simulink model "Symmetry_Inverter_imagined"  (Simulink 8.1)
settings: Solver=ode23t  StartTime=0.0  StopTime=tfin  RelTol=1e-4
values from neighbouring files (symbols this model uses):
  amp_feedback_saturation = 400    [Symmetry_ini_COPY.m]
  Butterworth_filter_order = 8    [Symmetry_ini_COPY.m]
  initial_value = [0.00,0.00,0.00,                  0,0,0]    [Symmetry_ini_COPY.m]
  k_symmetrcal_gain = 1e1    (= 10)    [Symmetry_ini_COPY.m]
  L_Network = [3.185e-3, 3.185e-3, 3.185e-3, 3.185e-3]    [Symmetry_ini_COPY.m]
  L_Source = [3.185e-3, 3.185e-3, 3.185e-3]    [Symmetry_ini_COPY.m]
  Load_R = [50,50,50]    [Symmetry_ini_COPY.m]
  Load_RL = [35.35,   35.35,   35.35;                   0.1125,  0.1125,  0.1125]    [Symmetry_ini_COPY.m]
  NetworkBreaker = [1e5,1e5,1e5,1e5]    [Symmetry_ini_COPY.m]
  P_gain = 5e-5    (= 5e-05)    [Symmetry_ini_COPY.m]
  phase_feedback_saturation = pi    (= 3.14159265359)    [Symmetry_ini_COPY.m]
  Phase_Source = [0,-2/3*pi,-4/3*pi]    [Symmetry_ini_COPY.m]
  PowerGain = [1e-5,1e-5,0]    [Symmetry_ini_COPY.m]
  PV_Power_Capacity = 5e3    (= 5000)    [Symmetry_ini_COPY.m]
  R_Source = [0.4, 0.4, 0.4]    [Symmetry_ini_COPY.m]
  sample = 10e-5    (= 0.0001)    [Symmetry_ini_COPY.m]    (also in animated_norms.m)
  Source_Frequency = [50,50,50]    [Symmetry_ini_COPY.m]
  Start_Control = 0.5    [Symmetry_ini_COPY.m]
  step_size = [1,1,1,                  0.08,0.08,0.08]    [Symmetry_ini_COPY.m]
  test_step = [0.5,0.5,0.5,                  0.02,0.02,0.02]    [Symmetry_ini_COPY.m]
  TransformerBreaker = [1e5,1e5,1e5;                     1e5,1e5,1e5]    [Symmetry_ini_COPY.m]
  Urms_Source = [230,230,230]    [Symmetry_ini_COPY.m]
undefined symbols (not defined in the file or in its folder): Capacitive_Load_RC, START_Load, Wire_resistence
libraries: powerlib x55, simulink x18, dspsigops x10, commsequence2 x6, powerlib_extras x6, dspxfrm3 x3, dsparch4 x3
(part 1 of 2)
settings Model: Creator=gorbep  LastModifiedBy=Neukirchner László
settings SolverCC: ZeroCrossAlgorithm=Adaptive  AlgebraicLoopSolver=LineSearch  SolverResetMethod=Robust
settings DataIOCC: SignalLoggingSaveFormat=Dataset
settings OptimizationCC: ExpressionDepthLimit=128  SimCompilerOptimization=On
settings DebuggingCC: UnderspecifiedInitializationDetection=Simplified  IgnoredZcDiagnostic=none  FcnCallInpInsideContextMsg=EnableAllAsError  StateNameClashWarn=none
settings GRTTargetCC: CodeReplacementLibrary=None  CombineOutputUpdateFcns=on  CPPClassGenCompliant=on  GRTInterface=off

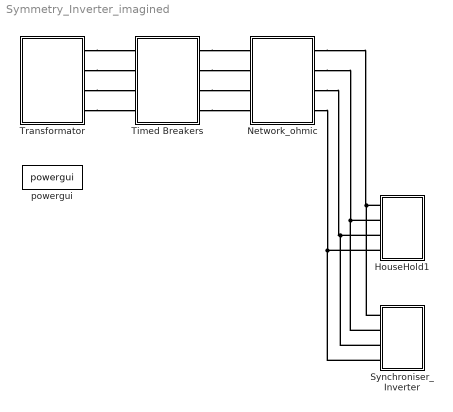
== system Symmetry_Inverter_imagined ==
  "HouseHold1 " : Subsystem
  Network_ohmic : Subsystem
  Synchroniser_Inverter : Subsystem
  Timed Breakers : Subsystem
  Transformator : Subsystem
  powergui : powerlib/powergui  SimulationMode=Continuous  SolverType=Tustin  SampleTime=50e-6  frequency=60  SPID=off  DisableSnubberDevices=off  DisableRonSwitches=off  DisableVfSwitches=off  SwTol=0  Interpol=off  DisplayEquations=off  frequencyindice=0  Pbase=100e6  ErrMax=1e-4  Iterations=50  UnitsV=kV  UnitsW=MW  FunctionMessages=off  echomessages=off  HookPort=off  EnableUseOfTLC=off  x0status=blocks  RestoreLinks=warning  ResistiveCurrentMeasurement=off  Frange=[0:2:500]  Ylog=off  Xlog=on  ShowGrid=off  save=off  variable=ZData  structure=0  ZoomFFT=on  StartTime=0.0  cycles=1  DisplayStyle=1  fundamental=60  FreqAxis=off  MaxFrequency=1000  frequencyindicesteady=1  RmsSteady=1  display=off  Ts=0  methode=off
  connections:
  Transformator/RConn1 -- Timed Breakers/LConn1
  Transformator/RConn2 -- Timed Breakers/LConn2
  Transformator/RConn3 -- Timed Breakers/LConn3
  Transformator/RConn4 -- Timed Breakers/LConn4
  Timed Breakers/RConn1 -- Network_ohmic/LConn1
  Timed Breakers/RConn3 -- Network_ohmic/LConn3
  Timed Breakers/RConn4 -- Network_ohmic/LConn4
  Timed Breakers/RConn2 -- Network_ohmic/LConn2
  Network_ohmic/RConn1 -- Synchroniser_Inverter/LConn1 -- "HouseHold1 "/LConn1
  Network_ohmic/RConn2 -- Synchroniser_Inverter/LConn2 -- "HouseHold1 "/LConn2
  Network_ohmic/RConn3 -- Synchroniser_Inverter/LConn3 -- "HouseHold1 "/LConn3
  Network_ohmic/RConn4 -- Synchroniser_Inverter/LConn4 -- "HouseHold1 "/LConn4

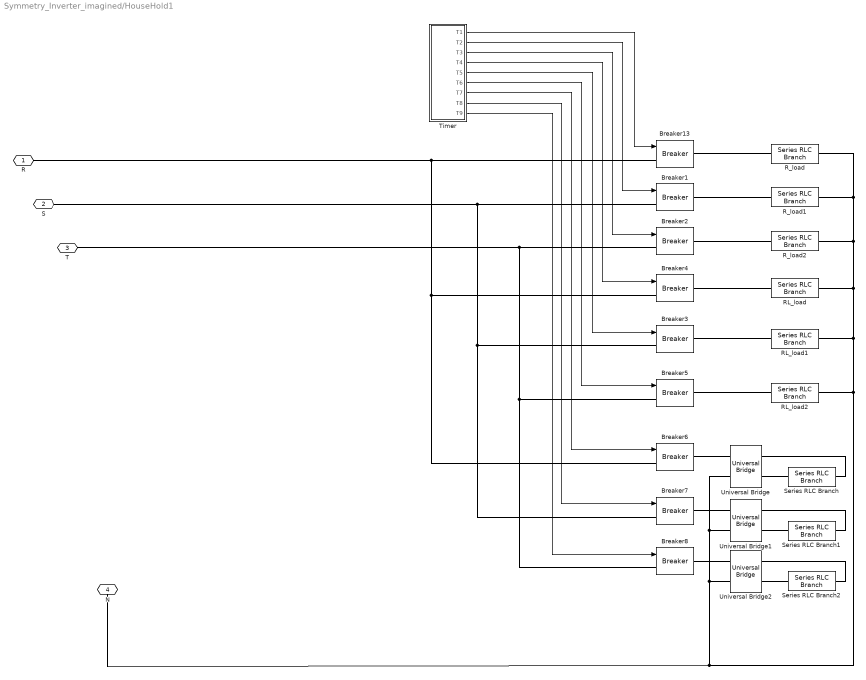
== system Symmetry_Inverter_imagined/HouseHold1  ==
  Breaker{1..8,13} (9 alike) : powerlib/Elements/Breaker  BreakerResistance=0.01  InitialState=0  SnubberResistance=1e7  SnubberCapacitance=inf  SwitchingTimes="[ 1/60  5/60 ]"  External=on  Measurements=None  MoreParameters=off  NoBreakLoop=off
  RL_load : powerlib/Elements/Series RLC Branch  LConnTagsString=__new0  RConnTagsString=__new0  BranchType=RL  Resistance=Load_RL(1,1)  Inductance=Load_RL(2,1)  SetiL0=off  InitialCurrent=0  Capacitance=1.0  Setx0=off  InitialVoltage=0  Measurements=None
  RL_load1 : powerlib/Elements/Series RLC Branch  LConnTagsString=__new0  RConnTagsString=__new0  BranchType=RL  Resistance=Load_RL(1,2)  Inductance=Load_RL(2,2)  SetiL0=off  InitialCurrent=0  Capacitance=1.0  Setx0=off  InitialVoltage=0  Measurements=None
  RL_load2 : powerlib/Elements/Series RLC Branch  LConnTagsString=__new0  RConnTagsString=__new0  BranchType=RL  Resistance=Load_RL(1,3)  Inductance=Load_RL(2,3)  SetiL0=off  InitialCurrent=0  Capacitance=1.0  Setx0=off  InitialVoltage=0  Measurements=None
  R_load : powerlib/Elements/Series RLC Branch  LConnTagsString=__new0  RConnTagsString=__new0  BranchType=R  Resistance=Load_R(1)  Inductance=0.003185  SetiL0=off  InitialCurrent=0  Capacitance=1.0  Setx0=off  InitialVoltage=0  Measurements=None
  R_load1 : powerlib/Elements/Series RLC Branch  LConnTagsString=__new0  RConnTagsString=__new0  BranchType=R  Resistance=Load_R(2)  Inductance=0.003185  SetiL0=off  InitialCurrent=0  Capacitance=1.0  Setx0=off  InitialVoltage=0  Measurements=None
  R_load2 : powerlib/Elements/Series RLC Branch  LConnTagsString=__new0  RConnTagsString=__new0  BranchType=R  Resistance=Load_R(3)  Inductance=0.003185  SetiL0=off  InitialCurrent=0  Capacitance=1.0  Setx0=off  InitialVoltage=0  Measurements=None
  Series RLC Branch : powerlib/Elements/Series RLC Branch  LConnTagsString=__new0  RConnTagsString=__new0  BranchType=RC  Resistance=Capacitive_Load_RC(1,1)  Inductance=1e-3  SetiL0=off  InitialCurrent=0  Capacitance=Capacitive_Load_RC(2,1)  Setx0=off  InitialVoltage=0  Measurements=None
  Series RLC Branch1 : powerlib/Elements/Series RLC Branch  LConnTagsString=__new0  RConnTagsString=__new0  BranchType=RC  Resistance=Capacitive_Load_RC(1,2)  Inductance=1e-3  SetiL0=off  InitialCurrent=0  Capacitance=Capacitive_Load_RC(2,2)  Setx0=off  InitialVoltage=0  Measurements=None
  Series RLC Branch2 : powerlib/Elements/Series RLC Branch  LConnTagsString=__new0  RConnTagsString=__new0  BranchType=RC  Resistance=Capacitive_Load_RC(1,3)  Inductance=1e-3  SetiL0=off  InitialCurrent=0  Capacitance=Capacitive_Load_RC(2,3)  Setx0=off  InitialVoltage=0  Measurements=None
  Timer : Subsystem
  Universal Bridge : powerlib/Power Electronics/Universal Bridge  Arms=2  SnubberResistance=1e5  SnubberCapacitance=inf  Device=Diodes  Ron=1e-3  Lon=0  ForwardVoltages="[  0  0  ]"  ForwardVoltage=0.8  GTOparameters=[ 10e-6 , 20e-6 ]  IGBTparameters=[ 1e-6 , 2e-6 ]  Measurements=None  Measurements_2=None  converterType=Rectifier
  Universal Bridge1 : powerlib/Power Electronics/Universal Bridge  Arms=2  SnubberResistance=1e5  SnubberCapacitance=inf  Device=Diodes  Ron=1e-3  Lon=0  ForwardVoltages="[  0  0  ]"  ForwardVoltage=0.8  GTOparameters=[ 10e-6 , 20e-6 ]  IGBTparameters=[ 1e-6 , 2e-6 ]  Measurements=None  Measurements_2=None  converterType=Rectifier
  Universal Bridge2 : powerlib/Power Electronics/Universal Bridge  Arms=2  SnubberResistance=1e5  SnubberCapacitance=inf  Device=Diodes  Ron=1e-3  Lon=0  ForwardVoltages="[  0  0  ]"  ForwardVoltage=0.8  GTOparameters=[ 10e-6 , 20e-6 ]  IGBTparameters=[ 1e-6 , 2e-6 ]  Measurements=None  Measurements_2=None  converterType=Rectifier
  R : PMIOPort  Port=1  Side=Left
  S : PMIOPort  Port=2  Side=Left
  T : PMIOPort  Port=3  Side=Left
  N : PMIOPort  Port=4  Side=Left
  wires:
  Timer/1(T1) -> Breaker13/1
  Timer/2(T2) -> Breaker1/1
  Timer/3(T3) -> Breaker2/1
  Timer/4(T4) -> Breaker4/1
  Timer/5(T5) -> Breaker3/1
  Timer/6(T6) -> Breaker5/1
  Timer/7(T7) -> Breaker6/1
  Timer/8(T8) -> Breaker7/1
  Timer/9(T9) -> Breaker8/1
  connections:
  R_load2/LConn1 -- Breaker2/RConn1
  R_load1/LConn1 -- Breaker1/RConn1
  Breaker13/RConn1 -- R_load/LConn1
  RL_load1/RConn1 -- RL_load/RConn1 -- R_load/RConn1 -- R_load1/RConn1 -- R_load2/RConn1 -- N/RConn1 -- Universal Bridge2/LConn2 -- Universal Bridge1/LConn2 -- Universal Bridge/LConn2 -- RL_load2/RConn1
  Breaker4/RConn1 -- RL_load/LConn1
  RL_load2/LConn1 -- Breaker5/RConn1
  RL_load1/LConn1 -- Breaker3/RConn1
  Breaker6/RConn1 -- Universal Bridge/LConn1
  Universal Bridge/RConn1 -- Series RLC Branch/LConn1
  Universal Bridge/RConn2 -- Series RLC Branch/RConn1
  Breaker7/RConn1 -- Universal Bridge1/LConn1
  Universal Bridge1/RConn2 -- Series RLC Branch1/RConn1
  Universal Bridge1/RConn1 -- Series RLC Branch1/LConn1
  Universal Bridge2/RConn2 -- Series RLC Branch2/RConn1
  Breaker8/RConn1 -- Universal Bridge2/LConn1
  Universal Bridge2/RConn1 -- Series RLC Branch2/LConn1
  Breaker6/LConn1 -- Breaker4/LConn1 -- R/RConn1 -- Breaker13/LConn1
  Breaker7/LConn1 -- Breaker3/LConn1 -- S/RConn1 -- Breaker1/LConn1
  Breaker8/LConn1 -- Breaker5/LConn1 -- T/RConn1 -- Breaker2/LConn1

== system Symmetry_Inverter_imagined/Network_ohmic ==
  Transf-L  Line -R1 : powerlib/Elements/Series RLC Branch  LConnTagsString=__new0  RConnTagsString=__new0  BranchType=R  Resistance=Wire_resistence  Inductance=L_Network(1)  SetiL0=off  InitialCurrent=0  Capacitance=1.0  Setx0=off  InitialVoltage=0  Measurements=None
  Transf-L  Line -R2 : powerlib/Elements/Series RLC Branch  LConnTagsString=__new0  RConnTagsString=__new0  BranchType=R  Resistance=Wire_resistence  Inductance=L_Network(2)  SetiL0=off  InitialCurrent=0  Capacitance=1.0  Setx0=off  InitialVoltage=0  Measurements=None
  Transf-L  Line -R3 : powerlib/Elements/Series RLC Branch  LConnTagsString=__new0  RConnTagsString=__new0  BranchType=R  Resistance=Wire_resistence  Inductance=L_Network(3)  SetiL0=off  InitialCurrent=0  Capacitance=1.0  Setx0=off  InitialVoltage=0  Measurements=None
  Transf-L  Line -R9 : powerlib/Elements/Series RLC Branch  LConnTagsString=__new0  RConnTagsString=__new0  BranchType=R  Resistance=Wire_resistence  Inductance=L_Network(4)  SetiL0=off  InitialCurrent=0  Capacitance=1.0  Setx0=off  InitialVoltage=0  Measurements=None
  R : PMIOPort  Port=1  Side=Left
  U : PMIOPort  Port=2  Side=Right
  S : PMIOPort  Port=3  Side=Left
  V : PMIOPort  Port=4  Side=Right
  T : PMIOPort  Port=5  Side=Left
  W : PMIOPort  Port=6  Side=Right
  N : PMIOPort  Port=7  Side=Left
  n : PMIOPort  Port=8  Side=Right
  connections:
  U/RConn1 -- Transf-L  Line -R1/RConn1
  V/RConn1 -- Transf-L  Line -R2/RConn1
  W/RConn1 -- Transf-L  Line -R3/RConn1
  Transf-L  Line -R3/LConn1 -- T/RConn1
  Transf-L  Line -R2/LConn1 -- S/RConn1
  R/RConn1 -- Transf-L  Line -R1/LConn1
  Transf-L  Line -R9/LConn1 -- N/RConn1
  n/RConn1 -- Transf-L  Line -R9/RConn1

== system Symmetry_Inverter_imagined/Synchroniser_Inverter ==
  Calculate_Norms : Subsystem
  Current Control : Subsystem
  NORM : Scope
      settings: ShowLegends=on  YMin=137464  YMax=137464  SaveName=ScopeData2
  Terminator{,1..5} (6 alike) : Terminator
  R : PMIOPort  Port=1  Side=Left
  S : PMIOPort  Port=2  Side=Left
  T : PMIOPort  Port=3  Side=Left
  N : PMIOPort  Port=4  Side=Left
  wires:
  Calculate_Norms/1(REG) -> Terminator/1
  Calculate_Norms/6(GEO) -> NORM/1, Current Control/1(NORM)
  Calculate_Norms/8(ANG) -> Current Control/2(ANG)
  Calculate_Norms/2(VEC_OLD) -> Terminator1/1
  Calculate_Norms/4(VEC_OLD_MEAN) -> Terminator3/1
  Calculate_Norms/7(GEO_MEAN) -> Terminator5/1
  Calculate_Norms/5(VEC_NEW_MEAN) -> Terminator4/1
  Calculate_Norms/3(VEC_NEW) -> Terminator2/1
  connections:
  R/RConn1 -- Current Control/RConn1 -- Calculate_Norms/LConn1
  S/RConn1 -- Current Control/RConn2 -- Calculate_Norms/LConn2
  T/RConn1 -- Current Control/RConn3 -- Calculate_Norms/LConn3
  N/RConn1 -- Current Control/RConn4 -- Calculate_Norms/LConn4

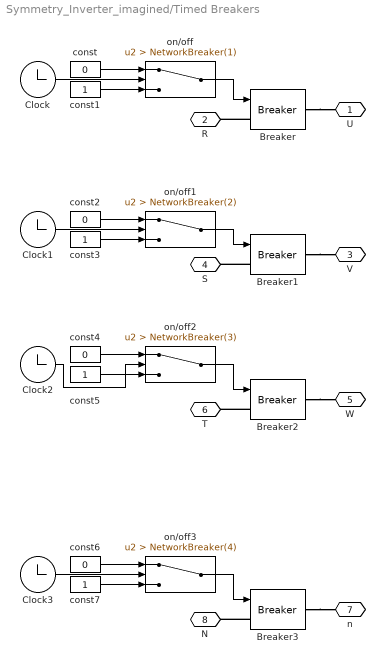
== system Symmetry_Inverter_imagined/Timed Breakers ==
  Breaker{,1..3} (4 alike) : powerlib/Elements/Breaker  BreakerResistance=0.01  InitialState=0  SnubberResistance=1e6  SnubberCapacitance=inf  SwitchingTimes="[1/60  5/60]"  External=on  Measurements=None  MoreParameters=on  NoBreakLoop=off
  Clock{,1..3} (4 alike) : Clock
      settings: Decimation=CLK
  const{,2,4,6} (4 alike) : Constant  Value=0
  const{1,3,5,7} (4 alike) : Constant
  on/off : Switch  Criteria=u2 > Threshold  Threshold=NetworkBreaker(1)
  on/off1 : Switch  Criteria=u2 > Threshold  Threshold=NetworkBreaker(2)
  on/off2 : Switch  Criteria=u2 > Threshold  Threshold=NetworkBreaker(3)
  on/off3 : Switch  Criteria=u2 > Threshold  Threshold=NetworkBreaker(4)
  U : PMIOPort  Port=1  Side=Right
  R : PMIOPort  Port=2  Side=Left
  V : PMIOPort  Port=3  Side=Right
  S : PMIOPort  Port=4  Side=Left
  W : PMIOPort  Port=5  Side=Right
  T : PMIOPort  Port=6  Side=Left
  n : PMIOPort  Port=7  Side=Right
  N : PMIOPort  Port=8  Side=Left
  wires:
  const/1 -> on/off/1
  const1/1 -> on/off/3
  Clock/1 -> on/off/2
  on/off/1 -> Breaker/1
  const2/1 -> on/off1/1
  const3/1 -> on/off1/3
  Clock1/1 -> on/off1/2
  const4/1 -> on/off2/1
  const5/1 -> on/off2/3
  Clock2/1 -> on/off2/2
  const6/1 -> on/off3/1
  const7/1 -> on/off3/3
  Clock3/1 -> on/off3/2
  on/off1/1 -> Breaker1/1
  on/off2/1 -> Breaker2/1
  on/off3/1 -> Breaker3/1
  connections:
  Breaker/RConn1 -- U/RConn1
  Breaker/LConn1 -- R/RConn1
  Breaker1/RConn1 -- V/RConn1
  Breaker1/LConn1 -- S/RConn1
  Breaker3/RConn1 -- n/RConn1
  Breaker3/LConn1 -- N/RConn1
  Breaker2/RConn1 -- W/RConn1
  Breaker2/LConn1 -- T/RConn1

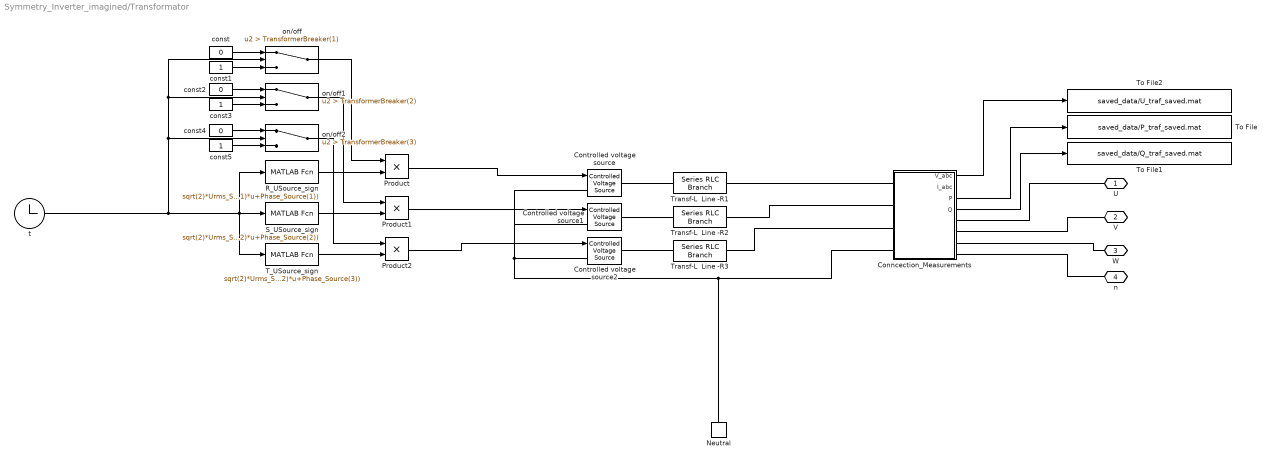
== system Symmetry_Inverter_imagined/Transformator ==
  " R_USource_sign" : MATLABFcn  MATLABFcn=sqrt(2)*Urms_Source(1)*sin(2*pi*Source_Frequency(1)*u+Phase_Source(1))  SampleTime=sample
  " S_USource_sign" : MATLABFcn  MATLABFcn=sqrt(2)*Urms_Source(2)*sin(2*pi*Source_Frequency(2)*u+Phase_Source(2))  SampleTime=sample
  " T_USource_sign" : MATLABFcn  MATLABFcn=sqrt(2)*Urms_Source(3)*sin(2*pi*Source_Frequency(2)*u+Phase_Source(3))  SampleTime=sample
  Conncection_Measurements : Subsystem
  Controlled voltage source : powerlib/Electrical Sources/Controlled Voltage Source  Initialize=off  Source_Type=AC  Amplitude=0  Phase=0  Frequency=0  Measurements=None
  Controlled voltage source1 : powerlib/Electrical Sources/Controlled Voltage Source  Initialize=off  Source_Type=AC  Amplitude=0  Phase=0  Frequency=0  Measurements=None
  Controlled voltage source2 : powerlib/Electrical Sources/Controlled Voltage Source  Initialize=off  Source_Type=AC  Amplitude=0  Phase=0  Frequency=0  Measurements=None
  Neutral : powerlib/Elements/Neutral  LConnTagsString=a  NodeNumber=10
  Product : Product
  Product1 : Product
  Product2 : Product
  To File : ToFile  Filename=saved_data/P_traf_saved.mat  MatrixName=P_traf_saved  SaveFormat=Timeseries  SampleTime=sample
  To File1 : ToFile  Filename=saved_data/Q_traf_saved.mat  MatrixName=Q_traf_saved  SaveFormat=Timeseries  SampleTime=sample
  To File2 : ToFile  Filename=saved_data/U_traf_saved.mat  MatrixName=U_traf_saved  SaveFormat=Timeseries  SampleTime=sample
  Transf-L  Line -R1 : powerlib/Elements/Series RLC Branch  LConnTagsString=__new0  RConnTagsString=__new0  BranchType=RL  Resistance=R_Source(1)  Inductance=L_Source(1)  SetiL0=off  InitialCurrent=0  Capacitance=1.0  Setx0=off  InitialVoltage=0  Measurements=None
  Transf-L  Line -R2 : powerlib/Elements/Series RLC Branch  LConnTagsString=__new0  RConnTagsString=__new0  BranchType=RL  Resistance=R_Source(2)  Inductance=L_Source(2)  SetiL0=off  InitialCurrent=0  Capacitance=1.0  Setx0=off  InitialVoltage=0  Measurements=None
  Transf-L  Line -R3 : powerlib/Elements/Series RLC Branch  LConnTagsString=__new0  RConnTagsString=__new0  BranchType=RL  Resistance=R_Source(3)  Inductance=L_Source(3)  SetiL0=off  InitialCurrent=0  Capacitance=1.0  Setx0=off  InitialVoltage=0  Measurements=None
  const : Constant  Value=0
  const1 : Constant
  const2 : Constant  Value=0
  const3 : Constant
  const4 : Constant  Value=0
  const5 : Constant
  on/off : Switch  Criteria=u2 > Threshold  Threshold=TransformerBreaker(1)
  on/off1 : Switch  Criteria=u2 > Threshold  Threshold=TransformerBreaker(2)
  on/off2 : Switch  Criteria=u2 > Threshold  Threshold=TransformerBreaker(3)
  t : Clock
      settings: Decimation=CLK
  U : PMIOPort  Port=1  Side=Right
  V : PMIOPort  Port=2  Side=Right
  W : PMIOPort  Port=3  Side=Right
  n : PMIOPort  Port=4  Side=Right
  wires:
  Conncection_Measurements/3(P) -> To File/1
  Conncection_Measurements/4(Q) -> To File1/1
  Conncection_Measurements/1(V_abc) -> To File2/1
  const/1 -> on/off/1
  const1/1 -> on/off/3
  t/1 -> " R_USource_sign"/1, " T_USource_sign"/1, " S_USource_sign"/1, on/off1/2, on/off/2, on/off2/2
  const2/1 -> on/off1/1
  const3/1 -> on/off1/3
  const4/1 -> on/off2/1
  const5/1 -> on/off2/3
  " T_USource_sign"/1 -> Product2/2
  " S_USource_sign"/1 -> Product1/2
  " R_USource_sign"/1 -> Product/2
  on/off/1 -> Product/1
  on/off1/1 -> Product1/1
  on/off2/1 -> Product2/1
  Product/1 -> Controlled voltage source/1
  Product1/1 -> Controlled voltage source1/1
  Product2/1 -> Controlled voltage source2/1
  connections:
  Neutral/LConn1 -- Conncection_Measurements/LConn4 -- Controlled voltage source/LConn1 -- Controlled voltage source1/LConn1 -- Controlled voltage source2/LConn1
  Transf-L  Line -R2/LConn1 -- Controlled voltage source1/RConn1
  Transf-L  Line -R3/LConn1 -- Controlled voltage source2/RConn1
  Transf-L  Line -R1/LConn1 -- Controlled voltage source/RConn1
  Conncection_Measurements/LConn1 -- Transf-L  Line -R1/RConn1
  Conncection_Measurements/LConn2 -- Transf-L  Line -R2/RConn1
  Conncection_Measurements/LConn3 -- Transf-L  Line -R3/RConn1
  U/RConn1 -- Conncection_Measurements/RConn1
  V/RConn1 -- Conncection_Measurements/RConn2
  W/RConn1 -- Conncection_Measurements/RConn3
  n/RConn1 -- Conncection_Measurements/RConn4

== system Symmetry_Inverter_imagined/HouseHold1 /Timer ==
  Clock : Clock
      settings: Decimation=CLK
  const : Constant
  const1 : Constant  Value=0
  on/off : Switch  Criteria=u2 > Threshold  Threshold=START_Load(1,1)
  on/off1 : Switch  Criteria=u2 > Threshold  Threshold=START_Load(1,2)
  on/off2 : Switch  Criteria=u2 > Threshold  Threshold=START_Load(1,3)
  on/off3 : Switch  Criteria=u2 > Threshold  Threshold=START_Load(2,1)
  on/off4 : Switch  Criteria=u2 > Threshold  Threshold=START_Load(2,2)
  on/off5 : Switch  Criteria=u2 > Threshold  Threshold=START_Load(2,3)
  on/off6 : Switch  Criteria=u2 > Threshold  Threshold=START_Load(3,1)
  on/off7 : Switch  Criteria=u2 > Threshold  Threshold=START_Load(3,2)
  on/off8 : Switch  Criteria=u2 > Threshold  Threshold=START_Load(3,3)
  T1 : Outport
  T2 : Outport  Port=2
  T3 : Outport  Port=3
  T4 : Outport  Port=4
  T5 : Outport  Port=5
  T6 : Outport  Port=6
  T7 : Outport  Port=7
  T8 : Outport  Port=8
  T9 : Outport  Port=9
  wires:
  on/off1/1 -> T2/1
  on/off/1 -> T1/1
  Clock/1 -> on/off8/2, on/off7/2, on/off6/2, on/off5/2, on/off4/2, on/off3/2, on/off2/2, on/off1/2, on/off/2
  on/off2/1 -> T3/1
  const1/1 -> on/off8/3, on/off7/3, on/off6/3, on/off5/3, on/off4/3, on/off3/3, on/off2/3, on/off1/3, on/off/3
  const/1 -> on/off8/1, on/off7/1, on/off6/1, on/off5/1, on/off4/1, on/off3/1, on/off2/1, on/off1/1, on/off/1
  on/off3/1 -> T4/1
  on/off4/1 -> T5/1
  on/off5/1 -> T6/1
  on/off6/1 -> T7/1
  on/off7/1 -> T8/1
  on/off8/1 -> T9/1

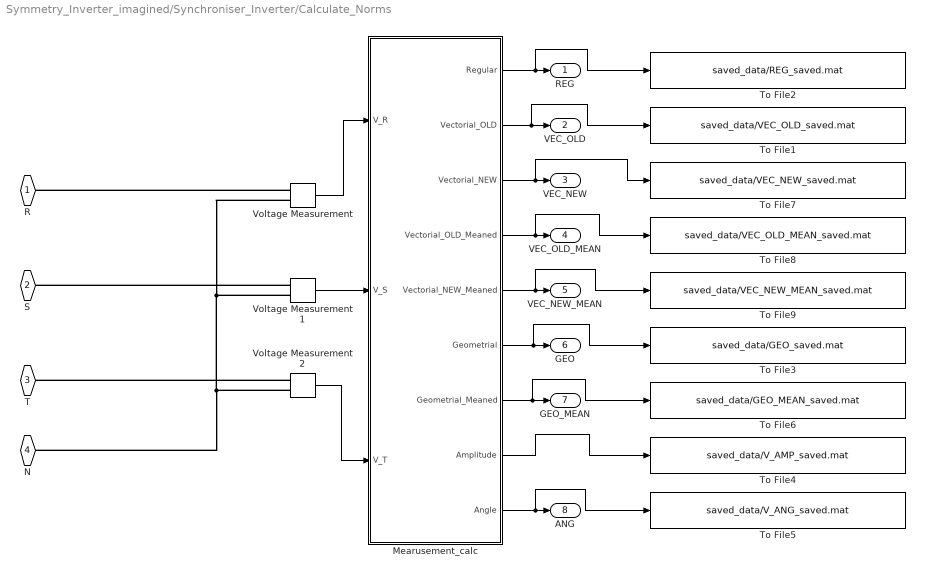
== system Symmetry_Inverter_imagined/Synchroniser_Inverter/Calculate_Norms ==
  Mearusement_calc : Subsystem
  To File1 : ToFile  Filename=saved_data/VEC_OLD_saved.mat  MatrixName=VEC_OLD_saved  SaveFormat=Timeseries  SampleTime=sample
  To File2 : ToFile  Filename=saved_data/REG_saved.mat  MatrixName=REG_saved  SaveFormat=Timeseries  SampleTime=sample
  To File3 : ToFile  Filename=saved_data/GEO_saved.mat  MatrixName=GEO_saved  SaveFormat=Timeseries  SampleTime=sample
  To File4 : ToFile  Filename=saved_data/V_AMP_saved.mat  MatrixName=V_AMP_saved  SaveFormat=Timeseries  SampleTime=sample
  To File5 : ToFile  Filename=saved_data/V_ANG_saved.mat  MatrixName=V_ANG_saved  SaveFormat=Timeseries  SampleTime=sample
  To File6 : ToFile  Filename=saved_data/GEO_MEAN_saved.mat  MatrixName=GEO_MEAN_saved  SaveFormat=Timeseries  SampleTime=sample
  To File7 : ToFile  Filename=saved_data/VEC_NEW_saved.mat  MatrixName=VEC_NEW_saved  SaveFormat=Timeseries  SampleTime=sample
  To File8 : ToFile  Filename=saved_data/VEC_OLD_MEAN_saved.mat  MatrixName=VEC_OLD_MEAN_saved  SaveFormat=Timeseries  SampleTime=sample
  To File9 : ToFile  Filename=saved_data/VEC_NEW_MEAN_saved.mat  MatrixName=VEC_NEW_MEAN_saved  SaveFormat=Timeseries  SampleTime=sample
  Voltage Measurement : powerlib/Measurements/Voltage Measurement  PhasorSimulation=off  OutputType=Complex  PSBequivalent=0
  Voltage Measurement1 : powerlib/Measurements/Voltage Measurement  PhasorSimulation=off  OutputType=Complex  PSBequivalent=0
  Voltage Measurement2 : powerlib/Measurements/Voltage Measurement  PhasorSimulation=off  OutputType=Complex  PSBequivalent=0
  R : PMIOPort  Port=1  Side=Left
  S : PMIOPort  Port=2  Side=Left
  T : PMIOPort  Port=3  Side=Left
  N : PMIOPort  Port=4  Side=Left
  REG : Outport
  VEC_OLD : Outport  Port=2
  VEC_NEW : Outport  Port=3
  VEC_OLD_MEAN : Outport  Port=4
  VEC_NEW_MEAN : Outport  Port=5
  GEO : Outport  Port=6
  GEO_MEAN : Outport  Port=7
  ANG : Outport  Port=8
  wires:
  Voltage Measurement/1 -> Mearusement_calc/1(V_R)
  Voltage Measurement1/1 -> Mearusement_calc/2(V_S)
  Voltage Measurement2/1 -> Mearusement_calc/3(V_T)
  Mearusement_calc/9(Angle) -> To File5/1, ANG/1
  Mearusement_calc/8(Amplitude) -> To File4/1
  Mearusement_calc/2(Vectorial_OLD) -> To File1/1, VEC_OLD/1
  Mearusement_calc/6(Geometrial) -> To File3/1, GEO/1
  Mearusement_calc/7(Geometrial_Meaned) -> To File6/1, GEO_MEAN/1
  Mearusement_calc/3(Vectorial_NEW) -> To File7/1, VEC_NEW/1
  Mearusement_calc/1(Regular) -> To File2/1, REG/1
  Mearusement_calc/4(Vectorial_OLD_Meaned) -> To File8/1, VEC_OLD_MEAN/1
  Mearusement_calc/5(Vectorial_NEW_Meaned) -> To File9/1, VEC_NEW_MEAN/1
  connections:
  Voltage Measurement2/LConn1 -- T/RConn1
  Voltage Measurement2/LConn2 -- Voltage Measurement/LConn2 -- Voltage Measurement1/LConn2 -- N/RConn1
  Voltage Measurement/LConn1 -- R/RConn1
  Voltage Measurement1/LConn1 -- S/RConn1

== system Symmetry_Inverter_imagined/Synchroniser_Inverter/Current Control ==
  NORM : Inport
  ANG : Inport  Port=2
  Current_Sources : Subsystem
  controller : Subsystem
  U : PMIOPort  Port=1  Side=Right
  V : PMIOPort  Port=2  Side=Right
  W : PMIOPort  Port=3  Side=Right
  n : PMIOPort  Port=4  Side=Right
  wires:
  NORM/1 -> controller/2(NORM)
  controller/1(Conteol_Current) -> Current_Sources/1(In1)
  Current_Sources/1(k) -> controller/1(k)
  ANG/1 -> controller/3(ANG)
  connections:
  n/RConn1 -- Current_Sources/RConn4
  U/RConn1 -- Current_Sources/RConn1
  V/RConn1 -- Current_Sources/RConn2
  W/RConn1 -- Current_Sources/RConn3

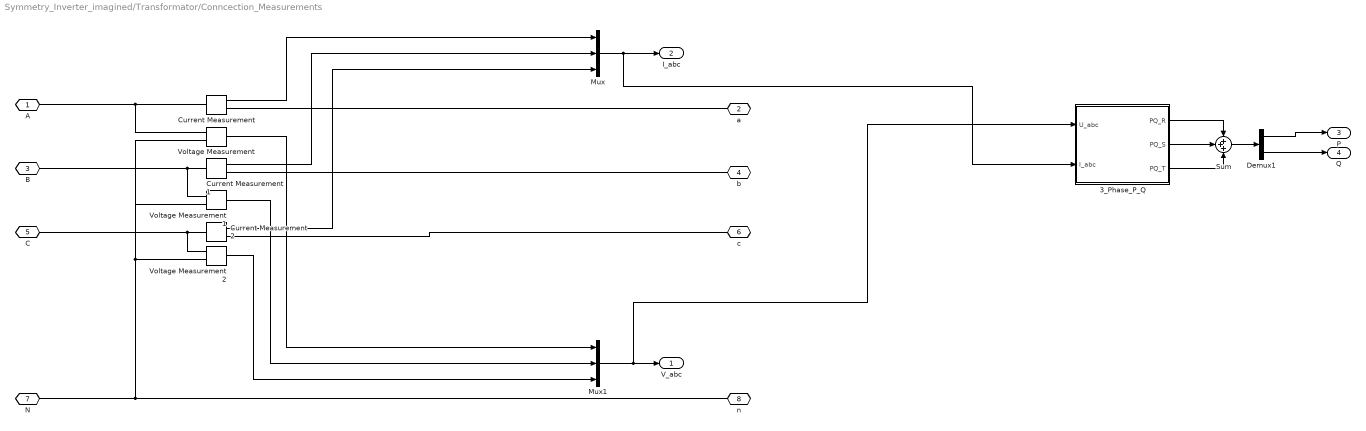
== system Symmetry_Inverter_imagined/Transformator/Conncection_Measurements ==
  3_Phase_P_Q : Subsystem
  Current Measurement : powerlib/Measurements/Current Measurement  PhasorSimulation=off  OutputType=Complex  PSBequivalent=0
  Current Measurement1 : powerlib/Measurements/Current Measurement  PhasorSimulation=off  OutputType=Complex  PSBequivalent=0
  Current Measurement2 : powerlib/Measurements/Current Measurement  PhasorSimulation=off  OutputType=Complex  PSBequivalent=0
  Demux1 : Demux  Outputs=2
  Mux : Mux  Inputs=3
  Mux1 : Mux  Inputs=3
  Sum : Sum  Inputs=+++
  Voltage Measurement : powerlib/Measurements/Voltage Measurement  PhasorSimulation=off  OutputType=Complex  PSBequivalent=0
  Voltage Measurement1 : powerlib/Measurements/Voltage Measurement  PhasorSimulation=off  OutputType=Complex  PSBequivalent=0
  Voltage Measurement2 : powerlib/Measurements/Voltage Measurement  PhasorSimulation=off  OutputType=Complex  PSBequivalent=0
  A : PMIOPort  Port=1  Side=Left
  a : PMIOPort  Port=2  Side=Right
  B : PMIOPort  Port=3  Side=Left
  b : PMIOPort  Port=4  Side=Right
  C : PMIOPort  Port=5  Side=Left
  c : PMIOPort  Port=6  Side=Right
  N : PMIOPort  Port=7  Side=Left
  n : PMIOPort  Port=8  Side=Right
  V_abc : Outport
  I_abc : Outport  Port=2
  P : Outport  Port=3
  Q : Outport  Port=4
  wires:
  Current Measurement1/1 -> Mux/2
  Current Measurement/1 -> Mux/1
  Voltage Measurement/1 -> Mux1/1
  Current Measurement2/1 -> Mux/3
  Voltage Measurement1/1 -> Mux1/2
  Voltage Measurement2/1 -> Mux1/3
  3_Phase_P_Q/2(PQ_S) -> Sum/2
  3_Phase_P_Q/1(PQ_R) -> Sum/1
  3_Phase_P_Q/3(PQ_T) -> Sum/3
  Mux/1 -> 3_Phase_P_Q/2(I_abc), I_abc/1
  Mux1/1 -> 3_Phase_P_Q/1(U_abc), V_abc/1
  Sum/1 -> Demux1/1
  Demux1/1 -> P/1
  Demux1/2 -> Q/1
  connections:
  Current Measurement2/RConn1 -- c/RConn1
  Current Measurement/RConn1 -- a/RConn1
  Current Measurement1/RConn1 -- b/RConn1
  Voltage Measurement2/LConn1 -- C/RConn1 -- Current Measurement2/LConn1
  Voltage Measurement2/LConn2 -- Voltage Measurement1/LConn2 -- Voltage Measurement/LConn2 -- N/RConn1 -- n/RConn1
  Voltage Measurement1/LConn1 -- B/RConn1 -- Current Measurement1/LConn1
  Voltage Measurement/LConn1 -- A/RConn1 -- Current Measurement/LConn1

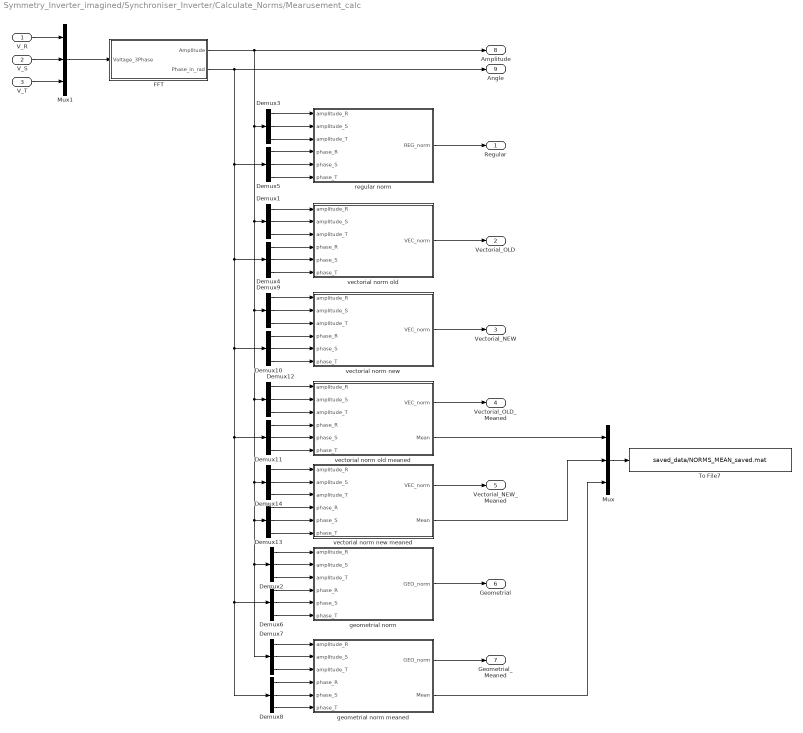
== system Symmetry_Inverter_imagined/Synchroniser_Inverter/Calculate_Norms/Mearusement_calc ==
  V_R : Inport
  V_S : Inport  Port=2
  V_T : Inport  Port=3
  Demux{1..14} (14 alike) : Demux  Outputs=3
  FFT : Subsystem
  Mux : Mux  Inputs=3
  Mux1 : Mux  Inputs=3
  To File7 : ToFile  Filename=saved_data/NORMS_MEAN_saved.mat  MatrixName=NORMS_MEAN_saved  SaveFormat=Timeseries  SampleTime=sample
  geometrial norm : MATLAB Function  TreatAsAtomicUnit=on
  geometrial norm meaned : MATLAB Function  TreatAsAtomicUnit=on
  regular norm : MATLAB Function  TreatAsAtomicUnit=on
  vectorial norm new : MATLAB Function  TreatAsAtomicUnit=on
  vectorial norm new meaned : MATLAB Function  TreatAsAtomicUnit=on
  vectorial norm old : MATLAB Function  TreatAsAtomicUnit=on
  vectorial norm old meaned : MATLAB Function  TreatAsAtomicUnit=on
  Regular : Outport
  Vectorial_OLD : Outport  Port=2
  Vectorial_NEW : Outport  Port=3
  Vectorial_OLD_Meaned : Outport  Port=4
  Vectorial_NEW_Meaned : Outport  Port=5
  Geometrial : Outport  Port=6
  Geometrial_Meaned : Outport  Port=7
  Amplitude : Outport  Port=8
  Angle : Outport  Port=9
  wires:
  V_R/1 -> Mux1/1
  V_T/1 -> Mux1/3
  Mux1/1 -> FFT/1(Voltage_3Phase)
  V_S/1 -> Mux1/2
  Demux1/1 -> vectorial norm old/1(amplitude_R)
  Demux1/2 -> vectorial norm old/2(amplitude_S)
  Demux1/3 -> vectorial norm old/3(amplitude_T)
  Demux4/1 -> vectorial norm old/4(phase_R)
  Demux4/2 -> vectorial norm old/5(phase_S)
  Demux4/3 -> vectorial norm old/6(phase_T)
  vectorial norm old/1(VEC_norm) -> Vectorial_OLD/1
  regular norm/1(REG_norm) -> Regular/1
  Demux3/1 -> regular norm/1(amplitude_R)
  Demux3/2 -> regular norm/2(amplitude_S)
  Demux3/3 -> regular norm/3(amplitude_T)
  Demux5/1 -> regular norm/4(phase_R)
  Demux5/2 -> regular norm/5(phase_S)
  Demux5/3 -> regular norm/6(phase_T)
  Demux2/1 -> geometrial norm/1(amplitude_R)
  Demux2/2 -> geometrial norm/2(amplitude_S)
  Demux2/3 -> geometrial norm/3(amplitude_T)
  Demux6/1 -> geometrial norm/4(phase_R)
  Demux6/2 -> geometrial norm/5(phase_S)
  Demux6/3 -> geometrial norm/6(phase_T)
  geometrial norm/1(GEO_norm) -> Geometrial/1
  Demux7/1 -> geometrial norm meaned/1(amplitude_R)
  Demux7/2 -> geometrial norm meaned/2(amplitude_S)
  Demux7/3 -> geometrial norm meaned/3(amplitude_T)
  Demux8/1 -> geometrial norm meaned/4(phase_R)
  Demux8/2 -> geometrial norm meaned/5(phase_S)
  Demux8/3 -> geometrial norm meaned/6(phase_T)
  geometrial norm meaned/1(GEO_norm) -> Geometrial_Meaned/1
  Demux9/1 -> vectorial norm new/1(amplitude_R)
  Demux9/2 -> vectorial norm new/2(amplitude_S)
  Demux9/3 -> vectorial norm new/3(amplitude_T)
  Demux10/1 -> vectorial norm new/4(phase_R)
  Demux10/2 -> vectorial norm new/5(phase_S)
  Demux10/3 -> vectorial norm new/6(phase_T)
  vectorial norm new/1(VEC_norm) -> Vectorial_NEW/1
  FFT/2(Phase_in_rad) -> Angle/1, Demux5/1, Demux4/1, Demux11/1, Demux6/1, Demux8/1, Demux10/1
  Demux12/1 -> vectorial norm old meaned/1(amplitude_R)
  Demux12/2 -> vectorial norm old meaned/2(amplitude_S)
  Demux12/3 -> vectorial norm old meaned/3(amplitude_T)
  Demux11/1 -> vectorial norm old meaned/4(phase_R)
  Demux11/2 -> vectorial norm old meaned/5(phase_S)
  Demux11/3 -> vectorial norm old meaned/6(phase_T)
  vectorial norm old meaned/1(VEC_norm) -> Vectorial_OLD_Meaned/1
  FFT/1(Amplitude) -> Amplitude/1, Demux3/1, Demux1/1, Demux12/1, Demux13/1, Demux2/1, Demux7/1, Demux14/1, Demux9/1
  Demux14/1 -> vectorial norm new meaned/1(amplitude_R)
  Demux14/2 -> vectorial norm new meaned/2(amplitude_S)
  Demux14/3 -> vectorial norm new meaned/3(amplitude_T)
  Demux13/1 -> vectorial norm new meaned/4(phase_R)
  Demux13/2 -> vectorial norm new meaned/5(phase_S)
  Demux13/3 -> vectorial norm new meaned/6(phase_T)
  vectorial norm new meaned/1(VEC_norm) -> Vectorial_NEW_Meaned/1
  Mux/1 -> To File7/1
  vectorial norm old meaned/2(Mean) -> Mux/1
  vectorial norm new meaned/2(Mean) -> Mux/2
  geometrial norm meaned/2(Mean) -> Mux/3

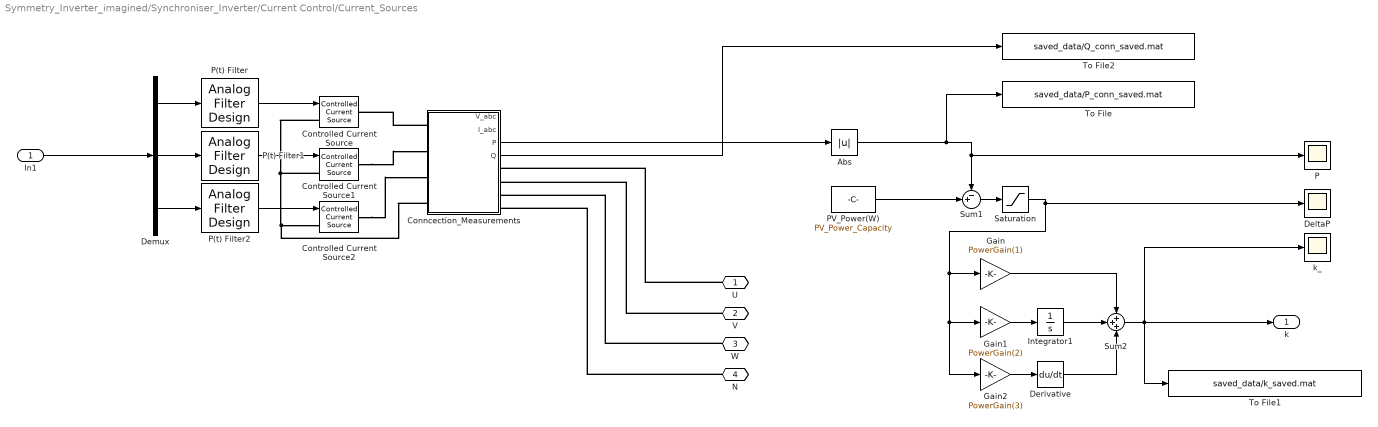
== system Symmetry_Inverter_imagined/Synchroniser_Inverter/Current Control/Current_Sources ==
  In1 : Inport
  Abs : Abs
  Conncection_Measurements : Subsystem
  Controlled Current Source : powerlib/Electrical Sources/Controlled Current Source  Initialize=on  Source_Type=AC  Amplitude=0  Phase=0  Frequency=0  Measurements=None
  Controlled Current Source1 : powerlib/Electrical Sources/Controlled Current Source  Initialize=on  Source_Type=AC  Amplitude=0  Phase=0  Frequency=0  Measurements=None
  Controlled Current Source2 : powerlib/Electrical Sources/Controlled Current Source  Initialize=on  Source_Type=AC  Amplitude=0  Phase=0  Frequency=0  Measurements=None
  DeltaP : Scope
      settings: YMin=5250  YMax=10000
  Demux : Demux  Outputs=3
  Derivative : Derivative
  Gain : Gain  Gain=PowerGain(1)
  Gain1 : Gain  Gain=PowerGain(2)
  Gain2 : Gain  Gain=PowerGain(3)
  Integrator1 : Integrator  InitialCondition=1
  P : Scope
      settings: YMin=0  YMax=27500  SaveName=ScopeData3
  P(t) Filter : dsparch4/Analog Filter Design  method=Butterworth  filttype=Lowpass  N=Butterworth_filter_order  Wlo=Butterworth_passband_frequency  Whi=80  Rp=2  Rs=40
  P(t) Filter1 : dsparch4/Analog Filter Design  method=Butterworth  filttype=Lowpass  N=Butterworth_filter_order  Wlo=Butterworth_passband_frequency  Whi=80  Rp=2  Rs=40
  P(t) Filter2 : dsparch4/Analog Filter Design  method=Butterworth  filttype=Lowpass  N=Butterworth_filter_order  Wlo=Butterworth_passband_frequency  Whi=80  Rp=2  Rs=40
  PV_Power(W) : Constant  Value=PV_Power_Capacity
  Saturation : Saturate  UpperLimit=inf  LowerLimit=0
  Sum1 : Sum  Inputs=-+|
  Sum2 : Sum  Inputs=+++
  To File : ToFile  Filename=saved_data/P_conn_saved.mat  MatrixName=P_conn_saved  SaveFormat=Timeseries  SampleTime=sample
  To File1 : ToFile  Filename=saved_data/k_saved.mat  MatrixName=k_saved  SaveFormat=Timeseries  SampleTime=sample
  To File2 : ToFile  Filename=saved_data/Q_conn_saved.mat  MatrixName=Q_conn_saved  SaveFormat=Timeseries  SampleTime=sample
  k_ : Scope
      settings: YMin=1  YMax=1.55
  U : PMIOPort  Port=1  Side=Right
  V : PMIOPort  Port=2  Side=Right
  W : PMIOPort  Port=3  Side=Right
  N : PMIOPort  Port=4  Side=Right
  k : Outport
  wires:
  In1/1 -> Demux/1
  Demux/1 -> P(t) Filter/1
  Demux/2 -> P(t) Filter1/1
  Demux/3 -> P(t) Filter2/1
  P(t) Filter/1 -> Controlled Current Source/1
  P(t) Filter1/1 -> Controlled Current Source1/1
  P(t) Filter2/1 -> Controlled Current Source2/1
  PV_Power(W)/1 -> Sum1/2
  Gain1/1 -> Integrator1/1
  Gain2/1 -> Derivative/1
  Integrator1/1 -> Sum2/2
  Gain/1 -> Sum2/1
  Derivative/1 -> Sum2/3
  Sum2/1 -> k_/1, To File1/1, k/1
  Sum1/1 -> Saturation/1
  Conncection_Measurements/3(P) -> Abs/1
  Conncection_Measurements/4(Q) -> To File2/1
  Abs/1 -> To File/1, Sum1/1, P/1
  Saturation/1 -> Gain2/1, Gain1/1, Gain/1, DeltaP/1
  connections:
  Controlled Current Source/LConn1 -- Controlled Current Source1/LConn1 -- Conncection_Measurements/LConn4 -- Controlled Current Source2/LConn1
  Conncection_Measurements/LConn1 -- Controlled Current Source/RConn1
  Controlled Current Source2/RConn1 -- Conncection_Measurements/LConn3
  U/RConn1 -- Conncection_Measurements/RConn1
  Controlled Current Source1/RConn1 -- Conncection_Measurements/LConn2
  N/RConn1 -- Conncection_Measurements/RConn4
  W/RConn1 -- Conncection_Measurements/RConn3
  V/RConn1 -- Conncection_Measurements/RConn2

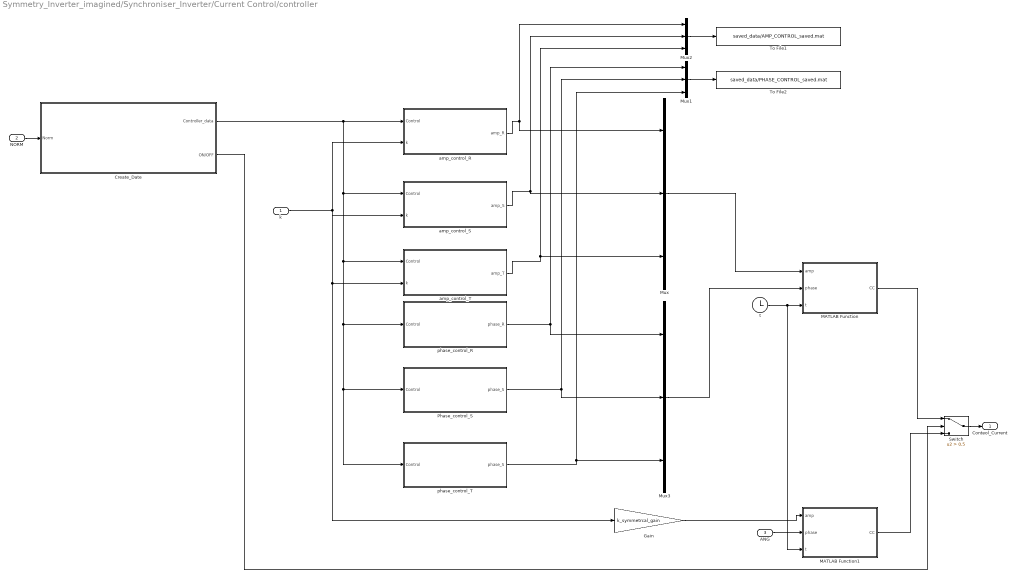
== system Symmetry_Inverter_imagined/Synchroniser_Inverter/Current Control/controller ==
  k : Inport
  NORM : Inport  Port=2
  ANG : Inport  Port=3
  Create_Date : Subsystem
  Gain : Gain  Gain=k_symmetrcal_gain
  MATLAB Function : MATLAB Function  TreatAsAtomicUnit=on
  MATLAB Function1 : MATLAB Function  TreatAsAtomicUnit=on
  Mux{,1..3} (4 alike) : Mux  Inputs=3
  Phase_control_S : Subsystem
  Switch : Switch  Criteria=u2 > Threshold  Threshold=0.5  InputSameDT=on
  To File1 : ToFile  Filename=saved_data/AMP_CONTROL_saved.mat  MatrixName=AMP_CONTROL_saved  SaveFormat=Timeseries  SampleTime=sample
  To File2 : ToFile  Filename=saved_data/PHASE_CONTROL_saved.mat  MatrixName=PHASE_CONTROL_saved  SaveFormat=Timeseries  SampleTime=sample
  amp_control_R : Subsystem
  amp_control_S : Subsystem
  amp_control_T : Subsystem
  phase_control_R : Subsystem
  phase_control_T : Subsystem
  t : Clock
      settings: Decimation=CLK
  Conteol_Current : Outport
  wires:
  amp_control_S/1(amp_S) -> Mux/2, Mux2/2
  amp_control_T/1(amp_T) -> Mux2/3, Mux/3
  Create_Date/1(Controller_data) -> phase_control_T/1(Control), Phase_control_S/1(Control), phase_control_R/1(Control), amp_control_T/1(Control), amp_control_S/1(Control), amp_control_R/1(Control)
  amp_control_R/1(amp_R) -> Mux/1, Mux2/1
  Phase_control_S/1(phase_S) -> Mux3/2, Mux1/2
  phase_control_T/1(phase_S) -> Mux3/3, Mux1/3
  Mux1/1 -> To File2/1
  phase_control_R/1(phase_R) -> Mux3/1, Mux1/1
  Mux2/1 -> To File1/1
  NORM/1 -> Create_Date/1(Norm)
  t/1 -> MATLAB Function1/3(t), MATLAB Function/3(t)
  MATLAB Function/1(CC) -> Switch/1
  Mux/1 -> MATLAB Function/1(amp)
  Mux3/1 -> MATLAB Function/2(phase)
  k/1 -> Gain/1, amp_control_T/2(k), amp_control_R/2(k), amp_control_S/2(k)
  ANG/1 -> MATLAB Function1/2(phase)
  Switch/1 -> Conteol_Current/1
  MATLAB Function1/1(CC) -> Switch/3
  Create_Date/2(ON/OFF) -> Switch/2
  Gain/1 -> MATLAB Function1/1(amp)

== system Symmetry_Inverter_imagined/Transformator/Conncection_Measurements/3_Phase_P_Q ==
  U_abc : Inport
  I_abc : Inport  Port=2
  Demux1 : Demux  Outputs=3
  Demux3 : Demux  Outputs=3
  P Q in3 : powerlib_extras/Measurements/Active & Reactive Power  f1=Source_Frequency(1)
  P Q in4 : powerlib_extras/Measurements/Active & Reactive Power  f1=Source_Frequency(2)
  P Q in5 : powerlib_extras/Measurements/Active & Reactive Power  f1=Source_Frequency(3)
  PQ_R : Outport
  PQ_S : Outport  Port=2
  PQ_T : Outport  Port=3
  wires:
  P Q in3/1 -> PQ_R/1
  P Q in4/1 -> PQ_S/1
  P Q in5/1 -> PQ_T/1
  Demux3/1 -> P Q in3/1
  Demux3/2 -> P Q in4/1
  Demux3/3 -> P Q in5/1
  Demux1/1 -> P Q in3/2
  Demux1/2 -> P Q in4/2
  Demux1/3 -> P Q in5/2
  U_abc/1 -> Demux3/1
  I_abc/1 -> Demux1/1

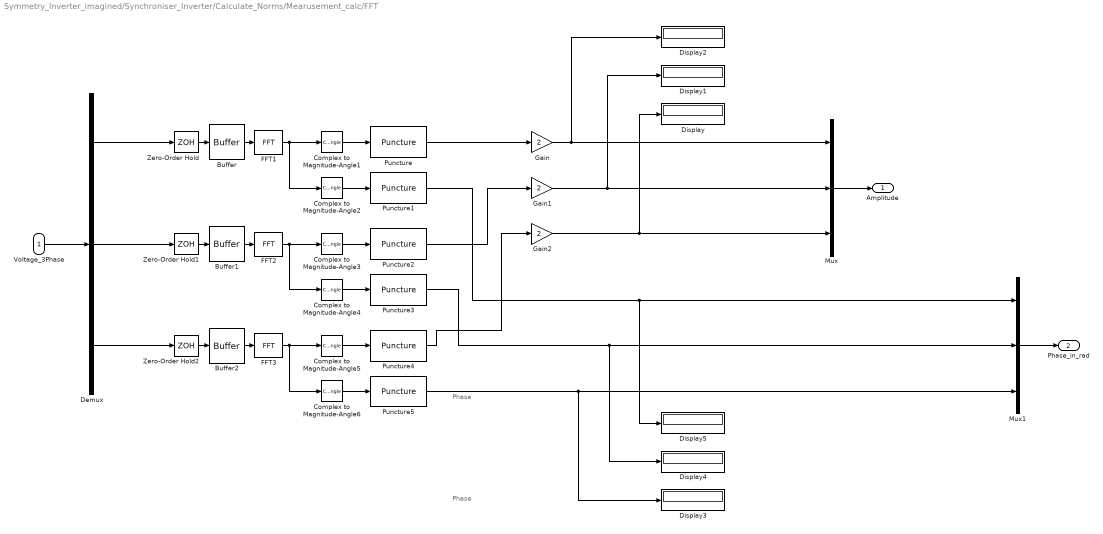
== system Symmetry_Inverter_imagined/Synchroniser_Inverter/Calculate_Norms/Mearusement_calc/FFT ==
  note: Phase
  note: Phase
  Voltage_3Phase : Inport
  Buffer : Buffer  N=128  TreatMby1Signals=One channel
  Buffer1 : Buffer  N=128  TreatMby1Signals=One channel
  Buffer2 : Buffer  N=128  TreatMby1Signals=One channel
  Complex to Magnitude-Angle1 : ComplexToMagnitudeAngle  Output=Magnitude
  Complex to Magnitude-Angle2 : ComplexToMagnitudeAngle  Output=Angle
  Complex to Magnitude-Angle3 : ComplexToMagnitudeAngle  Output=Magnitude
  Complex to Magnitude-Angle4 : ComplexToMagnitudeAngle  Output=Angle
  Complex to Magnitude-Angle5 : ComplexToMagnitudeAngle  Output=Magnitude
  Complex to Magnitude-Angle6 : ComplexToMagnitudeAngle  Output=Angle
  Demux : Demux  Outputs=3
  Display{,1..5} (6 alike) : Display
  FFT1 : dspxfrm3/FFT  CompMethod=Table lookup  TableOpt=NEW  TableOptActive=Speed  BitRevOrder=off  InheritFFTLength=on  FFTLength=64  RowConvenienceOn=on  FFTImplementation=Auto  SkipNorm=on  firstCoeffDataTypeStr=Inherit: Same word length as input  firstCoeffLastDataTypeStr=Inherit: Same word length as input  outputMin=[]  outputMax=[]  roundingMode=Floor  overflowMode=off
  FFT2 : dspxfrm3/FFT  CompMethod=Table lookup  TableOpt=NEW  TableOptActive=Speed  BitRevOrder=off  InheritFFTLength=on  FFTLength=64  RowConvenienceOn=on  FFTImplementation=Auto  SkipNorm=on  firstCoeffDataTypeStr=Inherit: Same word length as input  firstCoeffLastDataTypeStr=Inherit: Same word length as input  outputMin=[]  outputMax=[]  roundingMode=Floor  overflowMode=off
  FFT3 : dspxfrm3/FFT  CompMethod=Table lookup  TableOpt=NEW  TableOptActive=Speed  BitRevOrder=off  InheritFFTLength=on  FFTLength=64  RowConvenienceOn=on  FFTImplementation=Auto  SkipNorm=on  firstCoeffDataTypeStr=Inherit: Same word length as input  firstCoeffLastDataTypeStr=Inherit: Same word length as input  outputMin=[]  outputMax=[]  roundingMode=Floor  overflowMode=off
  Gain : Gain  Gain=2  SampleTime=sample
  Gain1 : Gain  Gain=2  SampleTime=sample
  Gain2 : Gain  Gain=2  SampleTime=sample
  Mux : Mux  Inputs=3
  Mux1 : Mux  Inputs=3
  Puncture{,1..5} (6 alike) : commsequence2/Puncture  punctureVector=s'
  Zero-Order Hold : ZeroOrderHold  SampleTime=20e-3/128
  Zero-Order Hold1 : ZeroOrderHold  SampleTime=20e-3/128
  Zero-Order Hold2 : ZeroOrderHold  SampleTime=20e-3/128
  Amplitude : Outport
  Phase_in_rad : Outport  Port=2
  wires:
  FFT1/1 -> Complex to Magnitude-Angle1/1, Complex to Magnitude-Angle2/1
  Buffer/1 -> FFT1/1
  Zero-Order Hold/1 -> Buffer/1
  Complex to Magnitude-Angle1/1 -> Puncture/1
  Complex to Magnitude-Angle2/1 -> Puncture1/1
  FFT2/1 -> Complex to Magnitude-Angle4/1, Complex to Magnitude-Angle3/1
  Buffer1/1 -> FFT2/1
  Zero-Order Hold1/1 -> Buffer1/1
  Complex to Magnitude-Angle3/1 -> Puncture2/1
  Complex to Magnitude-Angle4/1 -> Puncture3/1
  FFT3/1 -> Complex to Magnitude-Angle5/1, Complex to Magnitude-Angle6/1
  Buffer2/1 -> FFT3/1
  Zero-Order Hold2/1 -> Buffer2/1
  Complex to Magnitude-Angle5/1 -> Puncture4/1
  Complex to Magnitude-Angle6/1 -> Puncture5/1
  Voltage_3Phase/1 -> Demux/1
  Demux/2 -> Zero-Order Hold1/1
  Demux/3 -> Zero-Order Hold2/1
  Puncture/1 -> Gain/1
  Puncture2/1 -> Gain1/1
  Puncture4/1 -> Gain2/1
  Puncture1/1 -> Display5/1, Mux1/1
  Puncture3/1 -> Display4/1, Mux1/2
  Puncture5/1 -> Display3/1, Mux1/3
  Mux/1 -> Amplitude/1
  Mux1/1 -> Phase_in_rad/1
  Gain/1 -> Display2/1, Mux/1
  Gain1/1 -> Display1/1, Mux/2
  Gain2/1 -> Display/1, Mux/3
  Demux/1 -> Zero-Order Hold/1

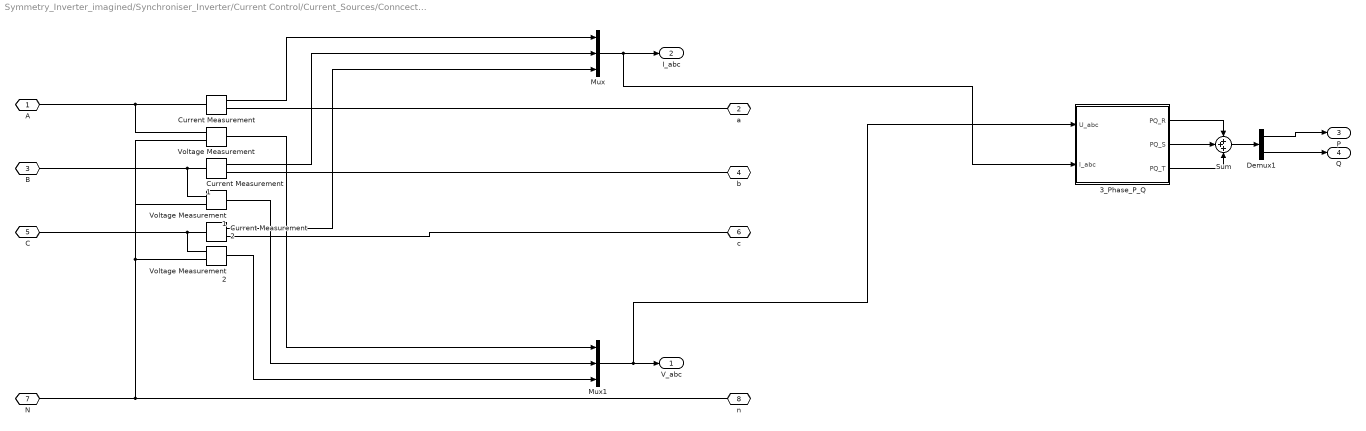
== system Symmetry_Inverter_imagined/Synchroniser_Inverter/Current Control/Current_Sources/Conncection_Measurements ==
  3_Phase_P_Q : Subsystem
  Current Measurement : powerlib/Measurements/Current Measurement  PhasorSimulation=off  OutputType=Complex  PSBequivalent=0
  Current Measurement1 : powerlib/Measurements/Current Measurement  PhasorSimulation=off  OutputType=Complex  PSBequivalent=0
  Current Measurement2 : powerlib/Measurements/Current Measurement  PhasorSimulation=off  OutputType=Complex  PSBequivalent=0
  Demux1 : Demux  Outputs=2
  Mux : Mux  Inputs=3
  Mux1 : Mux  Inputs=3
  Sum : Sum  Inputs=+++
  Voltage Measurement : powerlib/Measurements/Voltage Measurement  PhasorSimulation=off  OutputType=Complex  PSBequivalent=0
  Voltage Measurement1 : powerlib/Measurements/Voltage Measurement  PhasorSimulation=off  OutputType=Complex  PSBequivalent=0
  Voltage Measurement2 : powerlib/Measurements/Voltage Measurement  PhasorSimulation=off  OutputType=Complex  PSBequivalent=0
  A : PMIOPort  Port=1  Side=Left
  a : PMIOPort  Port=2  Side=Right
  B : PMIOPort  Port=3  Side=Left
  b : PMIOPort  Port=4  Side=Right
  C : PMIOPort  Port=5  Side=Left
  c : PMIOPort  Port=6  Side=Right
  N : PMIOPort  Port=7  Side=Left
  n : PMIOPort  Port=8  Side=Right
  V_abc : Outport
  I_abc : Outport  Port=2
  P : Outport  Port=3
  Q : Outport  Port=4
  wires:
  Current Measurement1/1 -> Mux/2
  Current Measurement/1 -> Mux/1
  Voltage Measurement/1 -> Mux1/1
  Current Measurement2/1 -> Mux/3
  Voltage Measurement1/1 -> Mux1/2
  Voltage Measurement2/1 -> Mux1/3
  3_Phase_P_Q/2(PQ_S) -> Sum/2
  3_Phase_P_Q/1(PQ_R) -> Sum/1
  3_Phase_P_Q/3(PQ_T) -> Sum/3
  Mux/1 -> 3_Phase_P_Q/2(I_abc), I_abc/1
  Mux1/1 -> 3_Phase_P_Q/1(U_abc), V_abc/1
  Sum/1 -> Demux1/1
  Demux1/1 -> P/1
  Demux1/2 -> Q/1
  connections:
  Current Measurement2/RConn1 -- c/RConn1
  Current Measurement/RConn1 -- a/RConn1
  Current Measurement1/RConn1 -- b/RConn1
  Voltage Measurement2/LConn1 -- C/RConn1 -- Current Measurement2/LConn1
  Voltage Measurement2/LConn2 -- Voltage Measurement1/LConn2 -- Voltage Measurement/LConn2 -- N/RConn1 -- n/RConn1
  Voltage Measurement1/LConn1 -- B/RConn1 -- Current Measurement1/LConn1
  Voltage Measurement/LConn1 -- A/RConn1 -- Current Measurement/LConn1

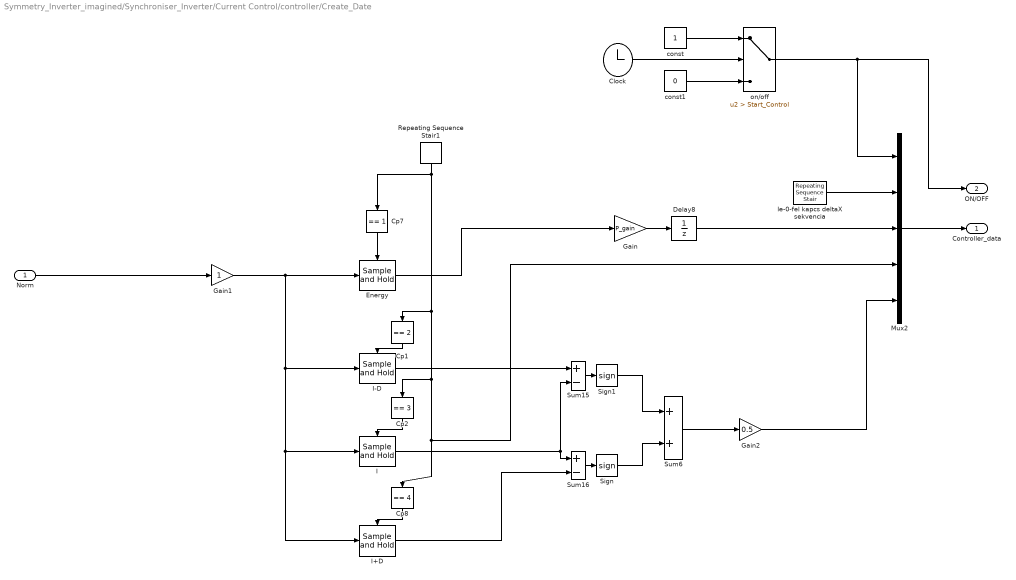
== system Symmetry_Inverter_imagined/Synchroniser_Inverter/Current Control/controller/Create_Date ==
  Norm : Inport
  Clock : Clock
      settings: Decimation=CLK
  Cp1 : simulink/Logic and Bit Operations/Compare To Constant  relop===  const=2  OutDataTypeStr=uint8  ZeroCross=off
  Cp2 : simulink/Logic and Bit Operations/Compare To Constant  relop===  const=3  OutDataTypeStr=uint8  ZeroCross=off
  Cp7 : simulink/Logic and Bit Operations/Compare To Constant  relop===  const=1  OutDataTypeStr=uint8  ZeroCross=off
  Cp8 : simulink/Logic and Bit Operations/Compare To Constant  relop===  const=4  OutDataTypeStr=uint8  ZeroCross=off
  Delay8 : UnitDelay  SampleTime=0.02
  Energy : dspsigops/Sample and Hold  trig=Rising edge  initCond=18  latchinput=off
  Gain : Gain  Gain=P_gain
  Gain1 : Gain
  Gain2 : Gain  Gain=0.5
  I : dspsigops/Sample and Hold  trig=Rising edge  initCond=0  latchinput=off
  I+D : dspsigops/Sample and Hold  trig=Rising edge  initCond=0  latchinput=off
  I-D : dspsigops/Sample and Hold  trig=Rising edge  initCond=0  latchinput=off
  Mux2 : Mux  Inputs=5
  Repeating Sequence Stair1 : simulink/Sources/Repeating Sequence Stair  OutValues=[1 2 3 4 5].'  tsamp=stair_sample  OutMin=[]  OutMax=[]  OutDataTypeStr=float('double')  OutputDataTypeScalingMode=Specify via dialog  OutDataType=float('double')  ConRadixGroup=Best Precision: Vector-wise  OutScaling=2^-12
  Sign : Signum
  Sign1 : Signum
  Sum15 : Sum  Inputs=+-
  Sum16 : Sum  Inputs=+-
  Sum6 : Sum
  const : Constant
  const1 : Constant  Value=0
  le-0-fel kapcs deltaX sekvencia : simulink/Sources/Repeating Sequence Stair  OutValues=[-1 0 1 0 0].'  tsamp=switch_sample  OutMin=[]  OutMax=[]  OutDataTypeStr=float('double')  OutputDataTypeScalingMode=Specify via dialog  OutDataType=float('double')  ConRadixGroup=Best Precision: Vector-wise  OutScaling=2^-12
  on/off : Switch  Criteria=u2 > Threshold  Threshold=Start_Control
  Controller_data : Outport
  ON/OFF : Outport  Port=2
  wires:
  Cp1/1 -> I-D/Trigger
  Repeating Sequence Stair1/1 -> Cp7/1, Mux2/4, Cp8/1, Cp2/1, Cp1/1
  Cp7/1 -> Energy/Trigger
  Energy/1 -> Gain/1
  Cp2/1 -> I/Trigger
  Cp8/1 -> I+D/Trigger
  Gain1/1 -> I+D/1, I/1, I-D/1, Energy/1
  I-D/1 -> Sum15/1
  I/1 -> Sum15/2, Sum16/1
  I+D/1 -> Sum16/2
  Sum16/1 -> Sign/1
  Sum15/1 -> Sign1/1
  Gain/1 -> Delay8/1
  Sign/1 -> Sum6/2
  Sign1/1 -> Sum6/1
  le-0-fel kapcs deltaX sekvencia/1 -> Mux2/2
  Delay8/1 -> Mux2/3
  on/off/1 -> Mux2/1, ON/OFF/1
  Mux2/1 -> Controller_data/1
  Norm/1 -> Gain1/1
  Sum6/1 -> Gain2/1
  const/1 -> on/off/1
  const1/1 -> on/off/3
  Clock/1 -> on/off/2
  Gain2/1 -> Mux2/5

== system Symmetry_Inverter_imagined/Synchroniser_Inverter/Current Control/controller/Phase_control_S ==
  Control : Inport
  Cp3 : simulink/Logic and Bit Operations/Compare To Constant  relop===  const=5  OutDataTypeStr=uint8  ZeroCross=off
  Delay : UnitDelay  SampleTime=0.001
  Delay4 : UnitDelay  SampleTime=0.02
  Demux2 : Demux  Outputs=5
  I Controller : dspsigops/Sample and Hold  trig=Rising edge  initCond=0  latchinput=off
  I3 Step : Constant  Value=step_size(5)
  "I3 init " : Constant  Value=initial_value(5)
  I3 test step : Constant  Value=test_step(5)
  Mask : simulink/Sources/Repeating Sequence Stair  OutValues=[0 0 0 0 1 0].'  tsamp=mask_sample  OutMin=[]  OutMax=[]  OutDataTypeStr=float('double')  OutputDataTypeScalingMode=Specify via dialog  OutDataType=float('double')  ConRadixGroup=Best Precision: Vector-wise  OutScaling=2^-12
  Product : Product  RndMeth=Zero
  Product12 : Product  RndMeth=Zero
  Product4 : Product  Inputs=4  RndMeth=Zero
  Product8 : Product  Inputs=4  RndMeth=Zero
  Saturation : Saturate  UpperLimit=phase_feedback_saturation  LowerLimit=-phase_feedback_saturation
  Sum : Sum  Inputs=|++
  Sum5 : Sum  Inputs=+++
  phase_S : Outport
  wires:
  Control/1 -> Demux2/1
  Product12/1 -> phase_S/1
  Product8/1 -> Sum/1
  Delay/1 -> Saturation/1
  "I3 init "/1 -> Sum5/2
  Delay4/1 -> Sum5/3
  Demux2/5 -> Product8/2
  Demux2/4 -> Product/2
  Demux2/3 -> Product4/3, Product8/1
  Demux2/2 -> Product4/2
  Demux2/1 -> Product12/1, Product8/4
  I3 Step/1 -> Product8/3
  Cp3/1 -> I Controller/Trigger
  Mask/1 -> Product/1, Product4/4
  Sum5/1 -> Product12/2
  I3 test step/1 -> Product4/1
  I Controller/1 -> Delay4/1, Delay/1
  Product4/1 -> Sum5/1
  Product/1 -> Cp3/1
  Sum/1 -> I Controller/1
  Saturation/1 -> Sum/2

== system Symmetry_Inverter_imagined/Synchroniser_Inverter/Current Control/controller/amp_control_R ==
  Control : Inport
  k : Inport  Port=2
  Cp3 : simulink/Logic and Bit Operations/Compare To Constant  relop===  const=5  OutDataTypeStr=uint8  ZeroCross=off
  Delay : UnitDelay  SampleTime=0.001
  Delay4 : UnitDelay  SampleTime=0.02
  Demux2 : Demux  Outputs=5
  I Controller : dspsigops/Sample and Hold  trig=Rising edge  initCond=0  latchinput=off
  I3 Step : Constant  Value=step_size(1)
  "I3 init " : Constant  Value=initial_value(1)
  I3 test step : Constant  Value=test_step(1)
  Mask : simulink/Sources/Repeating Sequence Stair  OutValues=[1 0 0 0 0 0].'  tsamp=mask_sample  OutMin=[]  OutMax=[]  OutDataTypeStr=float('double')  OutputDataTypeScalingMode=Specify via dialog  OutDataType=float('double')  ConRadixGroup=Best Precision: Vector-wise  OutScaling=2^-12
  Product : Product  RndMeth=Zero
  Product12 : Product  RndMeth=Zero
  Product4 : Product  Inputs=4  RndMeth=Zero
  Product8 : Product  Inputs=5  RndMeth=Zero
  Saturation : Saturate  UpperLimit=amp_feedback_saturation  LowerLimit=-amp_feedback_saturation
  Sum : Sum  Inputs=|++
  Sum5 : Sum  Inputs=+++
  amp_R : Outport
  wires:
  Control/1 -> Demux2/1
  Product12/1 -> amp_R/1
  Product8/1 -> Sum/1
  Delay/1 -> Saturation/1
  "I3 init "/1 -> Sum5/2
  Delay4/1 -> Sum5/3
  Demux2/5 -> Product8/2
  Demux2/4 -> Product/2
  Demux2/3 -> Product4/3, Product8/1
  Demux2/2 -> Product4/2
  Demux2/1 -> Product12/1, Product8/4
  I3 Step/1 -> Product8/3
  Cp3/1 -> I Controller/Trigger
  Mask/1 -> Product/1, Product4/4
  Sum5/1 -> Product12/2
  I3 test step/1 -> Product4/1
  I Controller/1 -> Delay4/1, Delay/1
  Product4/1 -> Sum5/1
  Product/1 -> Cp3/1
  Sum/1 -> I Controller/1
  Saturation/1 -> Sum/2
  k/1 -> Product8/5

== system Symmetry_Inverter_imagined/Synchroniser_Inverter/Current Control/controller/amp_control_S ==
  Control : Inport
  k : Inport  Port=2
  Cp3 : simulink/Logic and Bit Operations/Compare To Constant  relop===  const=5  OutDataTypeStr=uint8  ZeroCross=off
  Delay : UnitDelay  SampleTime=0.001
  Delay4 : UnitDelay  SampleTime=0.02
  Demux2 : Demux  Outputs=5
  I Controller : dspsigops/Sample and Hold  trig=Rising edge  initCond=0  latchinput=off
  I3 Step : Constant  Value=step_size(2)
  "I3 init " : Constant  Value=initial_value(2)
  I3 test step : Constant  Value=test_step(2)
  Mask : simulink/Sources/Repeating Sequence Stair  OutValues=[0 1 0 0 0 0].'  tsamp=mask_sample  OutMin=[]  OutMax=[]  OutDataTypeStr=float('double')  OutputDataTypeScalingMode=Specify via dialog  OutDataType=float('double')  ConRadixGroup=Best Precision: Vector-wise  OutScaling=2^-12
  Product : Product  RndMeth=Zero
  Product12 : Product  RndMeth=Zero
  Product4 : Product  Inputs=4  RndMeth=Zero
  Product8 : Product  Inputs=5  RndMeth=Zero
  Saturation : Saturate  UpperLimit=amp_feedback_saturation  LowerLimit=-amp_feedback_saturation
  Sum : Sum  Inputs=|++
  Sum5 : Sum  Inputs=+++
  amp_S : Outport
  wires:
  Saturation/1 -> Sum/2
  Sum/1 -> I Controller/1
  Product/1 -> Cp3/1
  Product4/1 -> Sum5/1
  I Controller/1 -> Delay/1, Delay4/1
  I3 test step/1 -> Product4/1
  Sum5/1 -> Product12/2
  Mask/1 -> Product4/4, Product/1
  Cp3/1 -> I Controller/Trigger
  I3 Step/1 -> Product8/3
  Demux2/1 -> Product8/4, Product12/1
  Demux2/2 -> Product4/2
  Demux2/3 -> Product8/1, Product4/3
  Demux2/4 -> Product/2
  Demux2/5 -> Product8/2
  Delay4/1 -> Sum5/3
  "I3 init "/1 -> Sum5/2
  Delay/1 -> Saturation/1
  Product8/1 -> Sum/1
  Product12/1 -> amp_S/1
  Control/1 -> Demux2/1
  k/1 -> Product8/5
